simulink model "sim1"  (R2015a)
settings: Solver=ode45  StartTime=0.0  StopTime=T  FixedStep=step  RelTol=1e-3
values from neighbouring files (symbols this model uses):
  b = 0    [lab2.m]
settings Model: Creator=Pedro  LastModifiedBy=abran

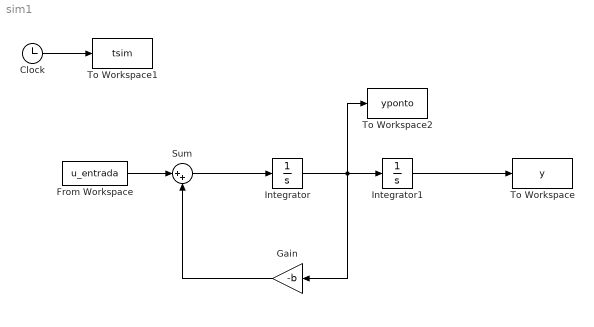
== system sim1 ==
  Clock : Clock
  From Workspace : FromWorkspace  VariableName=u_entrada  SampleTime=0
  Gain : Gain  Gain=-b
  Integrator : Integrator
  Integrator1 : Integrator  InitialCondition=1
  Sum : Sum  Inputs=|++
  To Workspace : ToWorkspace  VariableName=y  SampleTime=-1
  To Workspace1 : ToWorkspace  VariableName=tsim  SampleTime=-1
  To Workspace2 : ToWorkspace  VariableName=yponto  SampleTime=-1
  wires:
  Sum/1 -> Integrator/1
  Integrator/1 -> To Workspace2/1, Gain/1, Integrator1/1
  Integrator1/1 -> To Workspace/1
  Gain/1 -> Sum/2
  From Workspace/1 -> Sum/1
  Clock/1 -> To Workspace1/1
